simulink model "Q10_simulink"  (R2020b)
settings: Solver=VariableStepAuto  StartTime=0.0  StopTime=50  RelTol=1e-3
settings Model: Creator=User  LastModifiedBy=User

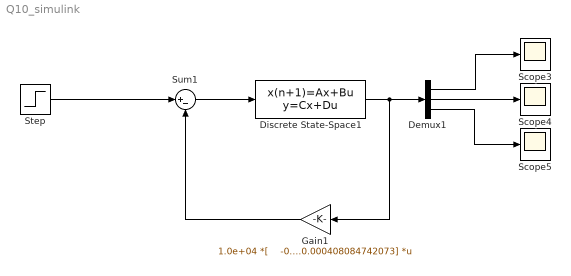
== system Q10_simulink ==
  Demux1 : Demux  Outputs=3
  Discrete State-Space1 : DiscreteStateSpace  A=|  B=|  C=[1 0 0; 0 1 0 ; 0 0 1]  D=[0;0;0]  InitialCondition=10  SampleTime=5
      A=|
      | [ 1.000000000000000 -21.150557534772830  -0.000604189555321
      |          ;          0   0.882496902584595   0.000048704536076
      |           ;         0                   0   0.630232382393690]
      B=|
      | [  -0.000088014915701
      |  ;  0.000011188695469
      |  ;  0.333725286648294]
  Gain1 : Gain  Gain=|  Multiplication=Matrix(K*u)
      | 1.0e+04 *[
      | 
      |    -0.217959452645970  8.571244823702385  0.000408084742073]
  Scope3 : Scope
  Scope4 : Scope
  Scope5 : Scope
  Step : Step  Time=0  SampleTime=0
  Sum1 : Sum  Inputs=|+-
  wires:
  Demux1/3 -> Scope5/1
  Demux1/2 -> Scope4/1
  Demux1/1 -> Scope3/1
  Step/1 -> Sum1/1
  Sum1/1 -> Discrete State-Space1/1
  Gain1/1 -> Sum1/2
  Discrete State-Space1/1 -> Gain1/1, Demux1/1
